simulink library "Vessel"  (R2023a)
settings: Solver=VariableStepAuto  StartTime=0.0  StopTime=10.0  RelTol=1e-3
undefined symbols (not defined in the file): A_ann_aor, alpha1, alpha2, atrium_ventricle, BSA, control, conversion_factor, DAP, DLVP, DP_close_aor, DP_open_aor, DPP, DRVP, E0, E_max, E_min, E_sa_0, E_sv_0, eta, g, K_vc_aor, K_vo_aor, l, L0, lambda, m1, m2, M_rg_aor, M_st_aor, MAP, MPP, n, P0, p_septum_on_off, p_th_on_off, phi, PVR, Q_max, rho, SAP, SI, sigma, SLVP, SPP, SRVP, SVR, t_delay, Ts, UVV_0, V0, V_0, V_max, V_tot, Y_aorta, Y_control
libraries: $bdroot x100, simulink x39, dspsigops x20, slpidlib x11, eeGeneralControl x2, dspstat3 x1
(part 3 of 4)

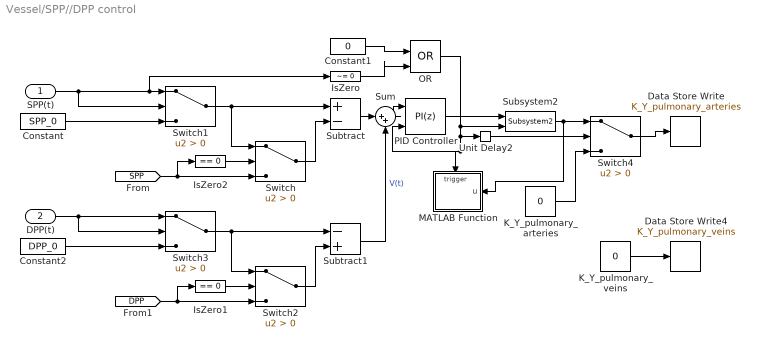
== system Vessel/SPP//DPP control ==
  SPP(t) : Inport
  DPP(t) : Inport  Port=2
  Constant : Constant  Value=SPP_0
  Constant1 : Constant  Value=0
  Constant2 : Constant  Value=DPP_0
  Data Store Write : DataStoreWrite  DataStoreName=K_Y_pulmonary_arteries  IndexOptions=Index vector (dialog)  Indices=1  OutputSizes=1
  Data Store Write4 : DataStoreWrite  DataStoreName=K_Y_pulmonary_veins  IndexOptions=Index vector (dialog)  Indices=1  OutputSizes=1
  IsZero : simulink/Logic and Bit Operations/Compare To Zero  relop=~=  OutDataTypeStr=boolean
      settings: LibrarySourceBlock=|
      | simulink/Quick Insert/Logic and Bit
      | Operations/IsZero
  IsZero1 : simulink/Logic and Bit Operations/Compare To Zero  relop===  OutDataTypeStr=boolean
      settings: LibrarySourceBlock=|
      | simulink/Quick Insert/Logic and Bit
      | Operations/IsZero
  IsZero2 : simulink/Logic and Bit Operations/Compare To Zero  relop===  OutDataTypeStr=boolean
      settings: LibrarySourceBlock=|
      | simulink/Quick Insert/Logic and Bit
      | Operations/IsZero
  K_Y_pulmonary_arteries : Constant  Value=0
  K_Y_pulmonary_veins : Constant  Value=0
  MATLAB Function : MATLAB Function  TreatAsAtomicUnit=on
  OR : Logic  Operator=OR  IconShape=distinctive  AllPortsSameDT=off  OutDataTypeStr=boolean
  PID Controller : slpidlib/PID Controller  Controller=PI  Form=Parallel  TimeDomain=Discrete-time  UseExternalTs=off  SampleTime=dt  IntegratorMethod=Forward Euler  FilterMethod=Forward Euler  ControllerParametersSource=internal  P=0.005  I=0.005  UseKiTs=off  D=0.01  N=100  UseFilter=on  TunerSelectOption=Transfer Function Based (PID Tuner App)  InitialConditionSource=internal  InitialConditionForIntegrator=0  InitialConditionForFilter=0  DifferentiatorICPrevScaledInput=0  ExternalReset=either  TrackingMode=off  Kt=1  LimitOutput=on  SatLimitsSource=internal  UpperSaturationLimit=2  LowerSaturationLimit=-0.99  LinearizeAsGain=on  AntiWindupMode=none  Kb=1  LimitIntegrator=off  UpperIntegratorSaturationLimit=inf  LowerIntegratorSaturationLimit=-inf  POutMin=[]  POutMax=[]  IOutMin=[]  IOutMax=[]  DOutMin=[]  DOutMax=[]  NOutMin=[]  NOutMax=[]  SumOutMin=[]  SumOutMax=[]  SaturationOutMin=[]  SaturationOutMax=[]  PParamMin=[]  PParamMax=[]  IParamMin=[]  IParamMax=[]  DParamMin=[]  DParamMax=[]  NParamMin=[]  NParamMax=[]  KbParamMin=[]  KbParamMax=[]  KtParamMin=[]  KtParamMax=[]  KbOutMin=[]  KbOutMax=[]  KtOutMin=[]  KtOutMax=[]  IntegratorOutMin=[]  IntegratorOutMax=[]  FilterOutMin=[]  FilterOutMax=[]  SumI1OutMin=[]  SumI1OutMax=[]  SumI2OutMin=[]  SumI2OutMax=[]  SumI3OutMin=[]  SumI3OutMax=[]  SumI4OutMin=[]  SumI4OutMax=[]  SumDOutMin=[]  SumDOutMax=[]  DifferentiatorOutMin=[]  DifferentiatorOutMax=[]  FilterDiffOutCoefMin=[]  FilterDiffOutCoefMax=[]  ReciprocalOutMin=[]  ReciprocalOutMax=[]  SumDenOutMin=[]  SumDenOutMax=[]  SumNumOutMin=[]  SumNumOutMax=[]  DivideOutMin=[]  DivideOutMax=[]  UdiffTsProdOutMin=[]  UdiffTsProdOutMax=[]  NTsProdOutMin=[]  NTsProdOutMax=[]  UintegralTsProdOutMin=[]  UintegralTsProdOutMax=[]  UngainTsProdOutMin=[]  UngainTsProdOutMax=[]  ClampingZeroOutDataTypeStr=Inherit: Inherit via back propagation  ClampingZeroOutMin=[]  ClampingZeroOutMax=[]  FilterDenConstantOutDataTypeStr=Inherit: Inherit via back propagation  FilterDenConstantOutMin=[]  FilterDenConstantOutMax=[]  PCopyOutDataTypeStr=Inherit: Inherit via back propagation  PCopyOutMin=[]  PCopyOutMax=[]  NCopyOutDataTypeStr=Inherit: Inherit via back propagation  NCopyOutMin=[]  NCopyOutMax=[]  IntegratorContinuousStateAttributes=''  IntegratorStateMustResolveToSignalObject=off  IntegratorRTWStateStorageClass=Auto  FilterContinuousStateAttributes=''  FilterStateMustResolveToSignalObject=off  FilterRTWStateStorageClass=Auto  ParallelPVariant=InternalParameters  IdealPVariant=Disabled  IVariant=InternalParameters  DVariant=Disabled  IntegratorVariant=Discrete  SatVariant=Enabled  AWVariant=Passthrough  PCopyVariant=Disabled  TRVariant=Disabled  FdbkBlocksVariant=Forward  IdealPFdbkVariant=Disabled  SatFdbkVariant=Disabled  DerivativeFilterVariant=Disabled  NVariant=Disabled  NCopyVariant=Disabled_SignalSpec  FilterICVariant=Disabled  IntegratorICVariant=InternalICs  ExternalResetVariant=ExternalReset  TRSumVariant=Passthrough  SumFdbkVariant=Disabled  SumVariant=Sum_PI  TsampFilterVariant=InternalTs  TsampNgainVariant=Passthrough  TsampIntegralVariant=Disabled_SignalSpec  ExternalSaturationOutDataTypeStr=Inherit: Same as second input
  Subsystem2 : $bdroot/SVR Control/Subsystem2  SystemSampleTime=-1  VariantActivationTime=update diagram  Latency=0  AutoFrameSizeCalculation=off
  Subtract : Sum  Inputs=+-
  Subtract1 : Sum  Inputs=-+
  Sum : Sum  Inputs=|++
  Switch{,1..4} (5 alike) : Switch  Criteria=u2 > Threshold  SaturateOnIntegerOverflow=off  InputSameDT=off
  Unit Delay2 : UnitDelay  SampleTime=-1  HasFrameUpgradeWarning=on
  wires:
  Sum/1 -> PID Controller/1
  Subtract/1 -> Sum/1
  Switch3/1 -> Subtract1/1, Switch2/1
  Constant2/1 -> Switch3/3
  Subtract1/1 -> Sum/2  "V(t)"
  IsZero1/1 -> Switch2/2
  Switch2/1 -> Subtract1/2
  DPP(t)/1 -> Switch3/2, Switch3/1
  [DPP] -> IsZero1/1, Switch2/3
  PID Controller/1 -> Subsystem2/1
  Constant1/1 -> OR/1
  IsZero/1 -> OR/2
  Switch1/1 -> Switch/1, Subtract/1
  SPP(t)/1 -> Switch1/1, IsZero/1, Switch1/2
  IsZero2/1 -> Switch/2
  Switch/1 -> Subtract/2
  [SPP] -> IsZero2/1, Switch/3
  Constant/1 -> Switch1/3
  Switch4/1 -> Data Store Write/1
  K_Y_pulmonary_veins/1 -> Data Store Write4/1
  K_Y_pulmonary_arteries/1 -> Switch4/3
  OR/1 -> Unit Delay2/1, PID Controller/2, MATLAB Function/Trigger, Subsystem2/2
  Subsystem2/1 -> Switch4/1, MATLAB Function/1(u)
  Unit Delay2/1 -> Switch4/2

== system Vessel/SRVP control ==
  SRVP(t) : Inport
  Constant : Constant  Value=SRVP_0
  Constant1 : Constant  Value=0
  Data Store Write : DataStoreWrite  DataStoreName=K_RV_Emax  IndexOptions=Index vector (dialog)  Indices=1  OutputSizes=1
  Data Store Write10 : DataStoreWrite  DataStoreName=K_RA_Emin  IndexOptions=Index vector (dialog)  Indices=1  OutputSizes=1
  Data Store Write11 : DataStoreWrite  DataStoreName=K_RV_Emin  IndexOptions=Index vector (dialog)  Indices=1  OutputSizes=1
  Data Store Write9 : DataStoreWrite  DataStoreName=K_RA_Emax  IndexOptions=Index vector (dialog)  Indices=1  OutputSizes=1
  IsZero : simulink/Logic and Bit Operations/Compare To Zero  relop=~=  OutDataTypeStr=boolean
      settings: LibrarySourceBlock=|
      | simulink/Quick Insert/Logic and Bit
      | Operations/IsZero
  IsZero2 : simulink/Logic and Bit Operations/Compare To Zero  relop===  OutDataTypeStr=boolean
      settings: LibrarySourceBlock=|
      | simulink/Quick Insert/Logic and Bit
      | Operations/IsZero
  K_RA_Emax : Constant  Value=0
  K_RA_Emin : Constant  Value=0
  K_RV_Emax : Constant  Value=0
  K_RV_Emin : Constant  Value=0
  MATLAB Function : MATLAB Function  TreatAsAtomicUnit=on
  OR : Logic  Operator=OR  IconShape=distinctive  AllPortsSameDT=off  OutDataTypeStr=boolean
  PID Controller : slpidlib/PID Controller  Controller=PI  Form=Parallel  TimeDomain=Discrete-time  UseExternalTs=off  SampleTime=dt  IntegratorMethod=Forward Euler  FilterMethod=Forward Euler  ControllerParametersSource=internal  P=0.005  I=0.005  UseKiTs=off  D=0.01  N=100  UseFilter=on  TunerSelectOption=Transfer Function Based (PID Tuner App)  InitialConditionSource=internal  InitialConditionForIntegrator=0  InitialConditionForFilter=0  DifferentiatorICPrevScaledInput=0  ExternalReset=either  TrackingMode=off  Kt=1  LimitOutput=on  SatLimitsSource=internal  UpperSaturationLimit=2  LowerSaturationLimit=-0.99  LinearizeAsGain=on  AntiWindupMode=none  Kb=1  LimitIntegrator=off  UpperIntegratorSaturationLimit=inf  LowerIntegratorSaturationLimit=-inf  POutMin=[]  POutMax=[]  IOutMin=[]  IOutMax=[]  DOutMin=[]  DOutMax=[]  NOutMin=[]  NOutMax=[]  SumOutMin=[]  SumOutMax=[]  SaturationOutMin=[]  SaturationOutMax=[]  PParamMin=[]  PParamMax=[]  IParamMin=[]  IParamMax=[]  DParamMin=[]  DParamMax=[]  NParamMin=[]  NParamMax=[]  KbParamMin=[]  KbParamMax=[]  KtParamMin=[]  KtParamMax=[]  KbOutMin=[]  KbOutMax=[]  KtOutMin=[]  KtOutMax=[]  IntegratorOutMin=[]  IntegratorOutMax=[]  FilterOutMin=[]  FilterOutMax=[]  SumI1OutMin=[]  SumI1OutMax=[]  SumI2OutMin=[]  SumI2OutMax=[]  SumI3OutMin=[]  SumI3OutMax=[]  SumI4OutMin=[]  SumI4OutMax=[]  SumDOutMin=[]  SumDOutMax=[]  DifferentiatorOutMin=[]  DifferentiatorOutMax=[]  FilterDiffOutCoefMin=[]  FilterDiffOutCoefMax=[]  ReciprocalOutMin=[]  ReciprocalOutMax=[]  SumDenOutMin=[]  SumDenOutMax=[]  SumNumOutMin=[]  SumNumOutMax=[]  DivideOutMin=[]  DivideOutMax=[]  UdiffTsProdOutMin=[]  UdiffTsProdOutMax=[]  NTsProdOutMin=[]  NTsProdOutMax=[]  UintegralTsProdOutMin=[]  UintegralTsProdOutMax=[]  UngainTsProdOutMin=[]  UngainTsProdOutMax=[]  ClampingZeroOutDataTypeStr=Inherit: Inherit via back propagation  ClampingZeroOutMin=[]  ClampingZeroOutMax=[]  FilterDenConstantOutDataTypeStr=Inherit: Inherit via back propagation  FilterDenConstantOutMin=[]  FilterDenConstantOutMax=[]  PCopyOutDataTypeStr=Inherit: Inherit via back propagation  PCopyOutMin=[]  PCopyOutMax=[]  NCopyOutDataTypeStr=Inherit: Inherit via back propagation  NCopyOutMin=[]  NCopyOutMax=[]  IntegratorContinuousStateAttributes=''  IntegratorStateMustResolveToSignalObject=off  IntegratorRTWStateStorageClass=Auto  FilterContinuousStateAttributes=''  FilterStateMustResolveToSignalObject=off  FilterRTWStateStorageClass=Auto  ParallelPVariant=InternalParameters  IdealPVariant=Disabled  IVariant=InternalParameters  DVariant=Disabled  IntegratorVariant=Discrete  SatVariant=Enabled  AWVariant=Passthrough  PCopyVariant=Disabled  TRVariant=Disabled  FdbkBlocksVariant=Forward  IdealPFdbkVariant=Disabled  SatFdbkVariant=Disabled  DerivativeFilterVariant=Disabled  NVariant=Disabled  NCopyVariant=Disabled_SignalSpec  FilterICVariant=Disabled  IntegratorICVariant=InternalICs  ExternalResetVariant=ExternalReset  TRSumVariant=Passthrough  SumFdbkVariant=Disabled  SumVariant=Sum_PI  TsampFilterVariant=InternalTs  TsampNgainVariant=Passthrough  TsampIntegralVariant=Disabled_SignalSpec  ExternalSaturationOutDataTypeStr=Inherit: Same as second input
  Subsystem2 : $bdroot/SVR Control/Subsystem2  SystemSampleTime=-1  VariantActivationTime=update diagram  Latency=0  AutoFrameSizeCalculation=off
  Subtract : Sum  Inputs=+-
  Switch : Switch  Criteria=u2 > Threshold  SaturateOnIntegerOverflow=off  InputSameDT=off
  Switch1 : Switch  Criteria=u2 > Threshold  SaturateOnIntegerOverflow=off  InputSameDT=off
  Switch2 : Switch  Criteria=u2 > Threshold  SaturateOnIntegerOverflow=off  InputSameDT=off
  Unit Delay2 : UnitDelay  SampleTime=-1  HasFrameUpgradeWarning=on
  wires:
  Subtract/1 -> PID Controller/1  "V(t)"
  Constant/1 -> Switch1/3
  [MPP] -> IsZero2/1, Switch/3
  Switch/1 -> Subtract/2
  IsZero2/1 -> Switch/2
  SRVP(t)/1 -> Switch1/2, IsZero/1, Switch1/1
  Switch1/1 -> Subtract/1, Switch/1
  IsZero/1 -> OR/2
  Constant1/1 -> OR/1
  PID Controller/1 -> Subsystem2/1
  K_RA_Emin/1 -> Data Store Write10/1
  K_RV_Emax/1 -> Switch2/3
  K_RV_Emin/1 -> Data Store Write11/1
  K_RA_Emax/1 -> Data Store Write9/1
  Switch2/1 -> Data Store Write/1
  OR/1 -> PID Controller/2, MATLAB Function/Trigger, Unit Delay2/1, Subsystem2/2
  Subsystem2/1 -> MATLAB Function/1(u), Switch2/1
  Unit Delay2/1 -> Switch2/2

== system Vessel/SVR Control ==
  SVR(t) : Inport
  Constant : Constant  Value=SVR_0
  Constant1 : Constant  Value=0
  Data Store Write : DataStoreWrite  DataStoreName=K_svr  IndexOptions=Index vector (dialog)  Indices=1  OutputSizes=1
  IsZero : simulink/Logic and Bit Operations/Compare To Zero  relop=~=  OutDataTypeStr=boolean
      settings: LibrarySourceBlock=|
      | simulink/Quick Insert/Logic and Bit
      | Operations/IsZero
  K_svr : Constant  Value=0
  MATLAB Function : MATLAB Function  TreatAsAtomicUnit=on
  OR : Logic  Operator=OR  IconShape=distinctive  AllPortsSameDT=off  OutDataTypeStr=boolean
  PID Controller : slpidlib/PID Controller  Controller=PI  Form=Parallel  TimeDomain=Continuous-time  UseExternalTs=off  SampleTime=-1  IntegratorMethod=Forward Euler  FilterMethod=Forward Euler  ControllerParametersSource=internal  P=0.2  I=0.2  UseKiTs=off  D=0.01  N=100  UseFilter=on  TunerSelectOption=Transfer Function Based (PID Tuner App)  InitialConditionSource=internal  InitialConditionForIntegrator=0  InitialConditionForFilter=0  DifferentiatorICPrevScaledInput=0  ExternalReset=either  TrackingMode=off  Kt=1  LimitOutput=off  SatLimitsSource=internal  UpperSaturationLimit=inf  LowerSaturationLimit=-inf  LinearizeAsGain=on  AntiWindupMode=none  Kb=1  LimitIntegrator=off  UpperIntegratorSaturationLimit=inf  LowerIntegratorSaturationLimit=-inf  POutMin=[]  POutMax=[]  IOutMin=[]  IOutMax=[]  DOutMin=[]  DOutMax=[]  NOutMin=[]  NOutMax=[]  SumOutMin=[]  SumOutMax=[]  SaturationOutMin=[]  SaturationOutMax=[]  PParamMin=[]  PParamMax=[]  IParamMin=[]  IParamMax=[]  DParamMin=[]  DParamMax=[]  NParamMin=[]  NParamMax=[]  KbParamMin=[]  KbParamMax=[]  KtParamMin=[]  KtParamMax=[]  KbOutMin=[]  KbOutMax=[]  KtOutMin=[]  KtOutMax=[]  IntegratorOutMin=[]  IntegratorOutMax=[]  FilterOutMin=[]  FilterOutMax=[]  SumI1OutMin=[]  SumI1OutMax=[]  SumI2OutMin=[]  SumI2OutMax=[]  SumI3OutMin=[]  SumI3OutMax=[]  SumI4OutMin=[]  SumI4OutMax=[]  SumDOutMin=[]  SumDOutMax=[]  DifferentiatorOutMin=[]  DifferentiatorOutMax=[]  FilterDiffOutCoefMin=[]  FilterDiffOutCoefMax=[]  ReciprocalOutMin=[]  ReciprocalOutMax=[]  SumDenOutMin=[]  SumDenOutMax=[]  SumNumOutMin=[]  SumNumOutMax=[]  DivideOutMin=[]  DivideOutMax=[]  UdiffTsProdOutMin=[]  UdiffTsProdOutMax=[]  NTsProdOutMin=[]  NTsProdOutMax=[]  UintegralTsProdOutMin=[]  UintegralTsProdOutMax=[]  UngainTsProdOutMin=[]  UngainTsProdOutMax=[]  ClampingZeroOutDataTypeStr=Inherit: Inherit via back propagation  ClampingZeroOutMin=[]  ClampingZeroOutMax=[]  FilterDenConstantOutDataTypeStr=Inherit: Inherit via back propagation  FilterDenConstantOutMin=[]  FilterDenConstantOutMax=[]  PCopyOutDataTypeStr=Inherit: Inherit via back propagation  PCopyOutMin=[]  PCopyOutMax=[]  NCopyOutDataTypeStr=Inherit: Inherit via back propagation  NCopyOutMin=[]  NCopyOutMax=[]  IntegratorContinuousStateAttributes=''  IntegratorStateMustResolveToSignalObject=off  IntegratorRTWStateStorageClass=Auto  FilterContinuousStateAttributes=''  FilterStateMustResolveToSignalObject=off  FilterRTWStateStorageClass=Auto  ParallelPVariant=InternalParameters  IdealPVariant=Disabled  IVariant=InternalParameters  DVariant=Disabled  IntegratorVariant=Continuous  SatVariant=Disabled  AWVariant=Passthrough  PCopyVariant=Disabled  TRVariant=Disabled  FdbkBlocksVariant=Forward  IdealPFdbkVariant=Disabled  SatFdbkVariant=Disabled  DerivativeFilterVariant=Disabled  NVariant=Disabled  NCopyVariant=Disabled_SignalSpec  FilterICVariant=Disabled  IntegratorICVariant=InternalICs  ExternalResetVariant=ExternalReset  TRSumVariant=Passthrough  SumFdbkVariant=Disabled  SumVariant=Sum_PI  TsampFilterVariant=InternalTs  TsampNgainVariant=Passthrough  TsampIntegralVariant=Disabled_SignalSpec  ExternalSaturationOutDataTypeStr=Inherit: Same as second input
  Subsystem1 : Subsystem
  Subsystem2 : Subsystem
  Subtract : Sum  Inputs=-+
  Switch : Switch  Criteria=u2 > Threshold  SaturateOnIntegerOverflow=off  InputSameDT=off
  Switch1 : Switch  Criteria=u2 > Threshold  SaturateOnIntegerOverflow=off  InputSameDT=off
  Switch2 : Switch  Criteria=u2 > Threshold  SaturateOnIntegerOverflow=off  InputSameDT=off
  Unit Delay : UnitDelay  SampleTime=-1  HasFrameUpgradeWarning=on
  wires:
  Subtract/1 -> PID Controller/1  "V(t)"
  Constant/1 -> Switch1/3
  [SVR] -> Subsystem1/1(In1), Switch/3
  Switch/1 -> Subtract/2
  Subsystem1/1(Out1) -> Switch/2
  SVR(t)/1 -> Switch1/2, IsZero/1, Switch1/1
  Switch1/1 -> Subtract/1, Switch/1
  IsZero/1 -> OR/2
  Constant1/1 -> OR/1
  Switch2/1 -> Data Store Write/1
  K_svr/1 -> Switch2/3
  OR/1 -> Subsystem2/2(Trigger), Unit Delay/1, PID Controller/2, MATLAB Function/Trigger
  PID Controller/1 -> Subsystem2/1(Signal)
  Subsystem2/1(Out) -> MATLAB Function/1(u), Switch2/1
  Unit Delay/1 -> Switch2/2

== system Vessel/Systolic Pressure ==
  P_in : Inport
  MinMax Running Resettable1 : simulink/Math Operations/MinMax Running Resettable  Function=max  vinit=0
      settings: AttributesFormatString=%<vinit>
  Pulse Generator1 : DiscretePulseGenerator  PulseType=Time based  TimeSource=Use external signal  Period=100  PulseWidth=1e-3
  Sample and Hold1 : dspsigops/Sample and Hold  trig=Rising edge  initCond=0  latchinput=on
  P_sys : Outport
  wires:
  MinMax Running Resettable1/1 -> Sample and Hold1/1
  Pulse Generator1/1 -> MinMax Running Resettable1/2, Sample and Hold1/Trigger
  Sample and Hold1/1 -> P_sys/1
  P_in/1 -> MinMax Running Resettable1/1
  [t_b] -> Pulse Generator1/1

== system Vessel/Time varying elastance (old) ==
  v_ed : Inport
  V : Inport  Port=2
  V' : Inport  Port=3
  Constant : Constant  Value=m1
  Constant1 : Constant  Value=m2
  Constant10 : Constant  Value=alpha2
  Constant12 : Constant  Value=Q_max
  Constant2 : Constant  Value=t_delay
  Constant4 : Constant  Value=E_max
  Constant5 : Constant  Value=E_min
  Constant6 : Constant  Value=sigma
  Constant7 : Constant  Value=alpha1
  Constant8 : Constant  Value=V_0
  Constant9 : Constant  Value=V_max
  Data Store Read : DataStoreRead  DataStoreName=T  IndexOptions=Index vector (dialog)  Indices=1  OutputSizes=1
  Data Store Read1 : DataStoreRead  DataStoreName=T  IndexOptions=Index vector (dialog)  Indices=1  OutputSizes=1
  Display : Display
  Display1 : Display
  MATLAB Function : MATLAB Function  TreatAsAtomicUnit=on
  Product : Product
  Sqrt : Sqrt
  E(t) : Outport
  wires:
  MATLAB Function/1(E) -> E(t)/1  "E(t)"
  Constant12/1 -> MATLAB Function/14(Q_max)
  v_ed/1 -> MATLAB Function/15(v_ed)
  V'/1 -> MATLAB Function/13(q)
  Constant9/1 -> MATLAB Function/12(V_max)
  Constant5/1 -> MATLAB Function/6(E_min)
  V/1 -> MATLAB Function/11(V)
  Constant8/1 -> MATLAB Function/10(V_0)
  Constant6/1 -> MATLAB Function/9(sigma)
  Data Store Read/1 -> MATLAB Function/8(T)
  Constant7/1 -> MATLAB Function/3(alpha1_ref)
  Constant/1 -> MATLAB Function/1(m1_ref)
  Constant4/1 -> MATLAB Function/5(E_max)
  [t_b] -> MATLAB Function/7(t)
  Constant1/1 -> MATLAB Function/2(m2_ref)
  Constant10/1 -> MATLAB Function/4(alpha2_ref)
  MATLAB Function/2(e_min) -> Display/1
  MATLAB Function/3(e_max) -> Display1/1
  Sqrt/1 -> Product/2
  Product/1 -> MATLAB Function/16(t_delay)
  Constant2/1 -> Product/1
  Data Store Read1/1 -> Sqrt/1

== system Vessel/Time varying elastance1 ==
  v_ed : Inport
  V : Inport  Port=2
  V' : Inport  Port=3
  Add : Sum
  Product : Product
  Subsystem : Subsystem
  e_max : Subsystem
  e_min : Subsystem
  k : Subsystem
  E(t) : Outport
  wires:
  Add/1 -> E(t)/1  "E(t)"
  e_max/1(e_max) -> k/3(e_max)
  Subsystem/2("f(g1, g2, t-t_delay)") -> Product/2
  k/1(k) -> Product/1
  Product/1 -> Add/1
  [t_b] -> Subsystem/1(t), k/1(t)
  V/1 -> e_min/1(V)
  e_min/1(e_min) -> Add/2, k/4(e_min)
  V'/1 -> e_max/2(V')
  v_ed/1 -> e_max/1(v_ed)
  Subsystem/1("f(g1, g2)") -> k/2("f(g1, g2)")

== system Vessel/Total Pulmonary resistance ==
  P_pu : Inport
  P_LA : Inport  Port=2
  Abs : Abs  SaturateOnIntegerOverflow=off
  Divide : Product  Inputs=*/
  Gain : Gain  Gain=60
  MAP1 : $bdroot/MAP  SystemSampleTime=-1  VariantActivationTime=update diagram  Latency=0  AutoFrameSizeCalculation=off
  Subtract1 : Sum  Inputs=-+
  tag scope: PVR=global
  wires:
  Abs/1 -> Gain/1
  Divide/1 -> Abs/1
  Subtract1/1 -> MAP1/1
  [CO] -> Divide/2
  P_LA/1 -> Subtract1/2
  Gain/1 -> [PVR]
  P_pu/1 -> Subtract1/1
  MAP1/1 -> Divide/1

== system Vessel/Total Systemic Resistance ==
  P_ao : Inport
  P_RA : Inport  Port=2
  Abs1 : Abs  SaturateOnIntegerOverflow=off
  Divide1 : Product  Inputs=*/
  Gain : Gain  Gain=60
  MAP1 : $bdroot/MAP  SystemSampleTime=-1  VariantActivationTime=update diagram  Latency=0  AutoFrameSizeCalculation=off
  Subtract1 : Sum  Inputs=+-
  tag scope: SVR=global
  wires:
  Abs1/1 -> Gain/1
  P_ao/1 -> Subtract1/1
  Divide1/1 -> Abs1/1
  Subtract1/1 -> MAP1/1
  P_RA/1 -> Subtract1/2
  [CO] -> Divide1/2
  Gain/1 -> [SVR]
  MAP1/1 -> Divide1/1

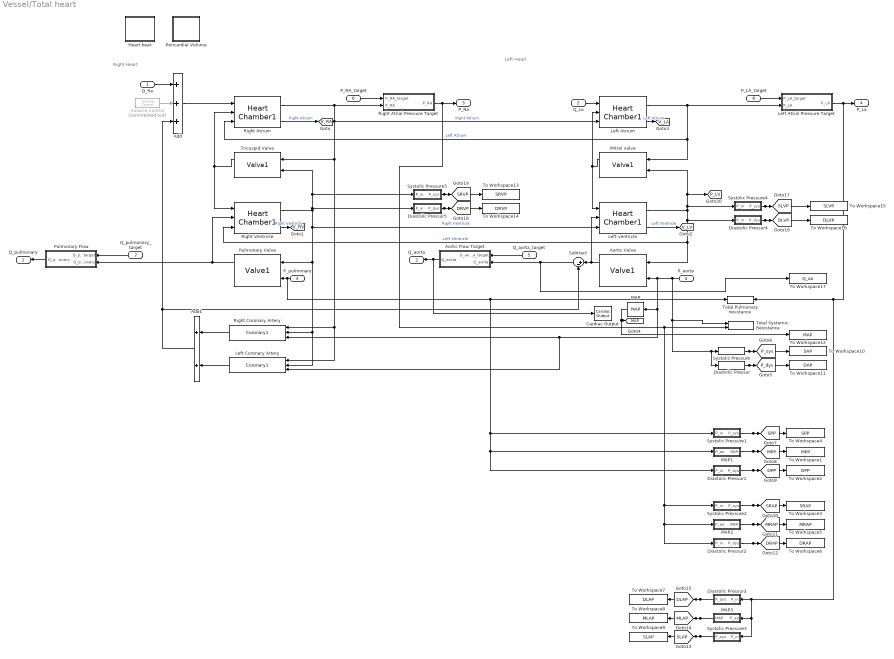
== system Vessel/Total heart ==
  note: Left Heart
  note: Right Heart
  Q_Ra : Inport
  Q_La : Inport  Port=2
  P_pulmonary : Inport  Port=3
  P_aorta : Inport  Port=4
  Q_aorta_target : Inport  Port=5
  P_RA_target : Inport  Port=6
  Q_pulmonary_target : Inport  Port=7
  P_LA_target : Inport  Port=8
  Add : Sum  Inputs=+++
  Add1 : Sum
  Aortic Flow Target : Subsystem
  Aortic Valve : $bdroot/Valve1  A_ann=A_ann_aor  K_vo=K_vo_aor  K_vc=K_vc_aor  M_st=M_st_aor  M_rg=M_rg_aor  DP_open=DP_open_aor  DP_close=DP_close_aor  Q_max=Q_max_lv  Q_min=-1000
  Cardiac Output : $bdroot/Cardiac Output  SystemSampleTime=-1  VariantActivationTime=update diagram  Latency=0  AutoFrameSizeCalculation=off
  Diastolic Pressur : $bdroot/Diastolic Pressur  SystemSampleTime=-1  VariantActivationTime=update diagram  Latency=0  AutoFrameSizeCalculation=off
  Diastolic Pressur1 : Subsystem
  Diastolic Pressur2 : Subsystem
  Diastolic Pressur3 : Subsystem
  Diastolic Pressur4 : Subsystem
  Diastolic Pressur5 : Subsystem
  Heart beat : Subsystem
  Left Atrial Pressure Target : Subsystem
  Left Atrium : $bdroot/Heart Chamber1  control=Left Atrium  E_max=E_max_la  E_min=E_min_la  alpha1=alpha1_la  alpha2=alpha2_la  m1=m1_la  m2=m2_la  R_wall=R_wall_la  t_delay=t_delay_la  V_0=V_0_la  v_o=v_o_la  sigma=sigma_la  V_max=V_max_la  Q_max=Q_max_la  T0=T0  P_pc_0=P_pc_0  K_pc=K_pc  V_pc_0=V_pc_0  V_pe=V_pe  phi_pc=phi_pc  E_sa_0=E_sa_0  E_sv_0=E_sv_0  atrium_ventricle=Atrium
  Left Coronary Artery : $bdroot/Coronary1  R_ca=R_lca
  Left ventricle : $bdroot/Heart Chamber1  control=Left Ventricle  E_max=E_max_lv  E_min=E_min_lv  alpha1=alpha1_lv  alpha2=alpha2_lv  m1=m1_lv  m2=m2_lv  R_wall=R_wall_lv  t_delay=t_delay_lv  V_0=V_0_lv  v_o=v_o_lv  sigma=sigma_lv  V_max=V_max_lv  Q_max=Q_max_lv  T0=T0  P_pc_0=P_pc_0  K_pc=K_pc  V_pc_0=V_pc_0  V_pe=V_pe  phi_pc=phi_pc  E_sa_0=E_sa_0  E_sv_0=E_sv_0  atrium_ventricle=Ventricle
  MAP : $bdroot/MAP  SystemSampleTime=-1  VariantActivationTime=update diagram  Latency=0  AutoFrameSizeCalculation=off
  MAP1 : Subsystem
  MAP2 : Subsystem
  MAP3 : Subsystem
  Mitral valve : $bdroot/Valve1  A_ann=A_ann_mit  K_vo=K_vo_mit  K_vc=K_vc_mit  M_st=M_st_mit  M_rg=M_rg_mit  DP_open=DP_open_mit  DP_close=DP_close_mit  Q_max=Q_max_la  Q_min=-1000
  Pericardial Volume : Subsystem
  Pulmonary Flow : Subsystem
  Pulmonary Valve : $bdroot/Valve1  A_ann=A_ann_pul  K_vo=K_vo_pul  K_vc=K_vc_pul  M_st=M_st_pul  M_rg=M_rg_pul  DP_open=DP_open_pul  DP_close=DP_close_pul  Q_max=Q_max_rv  Q_min=-1000
  Right Atrial Pressure Target : Subsystem
  Right Atrium : $bdroot/Heart Chamber1  control=Right Atrium  E_max=E_max_ra  E_min=E_min_ra  alpha1=alpha1_ra  alpha2=alpha2_ra  m1=m1_ra  m2=m2_ra  R_wall=R_wall_ra  t_delay=t_delay_ra  V_0=V_0_ra  v_o=v_o_ra  sigma=sigma_ra  V_max=V_max_ra  Q_max=Q_max_ra  T0=T0  P_pc_0=P_pc_0  K_pc=K_pc  V_pc_0=V_pc_0  V_pe=V_pe  phi_pc=phi_pc  E_sa_0=E_sa_0  E_sv_0=E_sv_0  atrium_ventricle=Atrium
  Right Coronary Artery : $bdroot/Coronary1  R_ca=R_rca
  Right Ventricle : $bdroot/Heart Chamber1  control=Right Ventricle  E_max=E_max_rv  E_min=E_min_rv  alpha1=alpha1_rv  alpha2=alpha2_rv  m1=m1_rv  m2=m2_rv  R_wall=R_wall_rv  t_delay=t_delay_rv  V_0=V_0_rv  v_o=v_o_rv  sigma=sigma_rv  V_max=V_max_rv  Q_max=Q_max_rv  T0=T0  P_pc_0=P_pc_0  K_pc=K_pc  V_pc_0=V_pc_0  V_pe=V_pe  phi_pc=phi_pc  E_sa_0=E_sa_0  E_sv_0=E_sv_0  atrium_ventricle=Ventricle
  Subtract : Sum  Inputs=|+-
  Systolic Pressure : $bdroot/Systolic Pressure  SystemSampleTime=-1  VariantActivationTime=update diagram  Latency=0  AutoFrameSizeCalculation=off
  Systolic Pressure1 : Subsystem
  Systolic Pressure2 : Subsystem
  Systolic Pressure3 : Subsystem
  Systolic Pressure4 : Subsystem
  Systolic Pressure5 : Subsystem
  To Workspace1 : ToWorkspace  VariableName=MPP  SampleTime=-1
  To Workspace10 : ToWorkspace  VariableName=SAP  SampleTime=-1
  To Workspace11 : ToWorkspace  VariableName=DAP  SampleTime=-1
  To Workspace12 : ToWorkspace  VariableName=MAP  SampleTime=-1
  To Workspace13 : ToWorkspace  VariableName=SRVP  SampleTime=-1
  To Workspace14 : ToWorkspace  VariableName=DRVP  SampleTime=-1
  To Workspace15 : ToWorkspace  VariableName=SLVP  SampleTime=-1
  To Workspace16 : ToWorkspace  VariableName=DLVP  SampleTime=-1
  To Workspace17 : ToWorkspace  VariableName=Q_ao  SampleTime=-1
  To Workspace2 : ToWorkspace  VariableName=DPP  SampleTime=-1
  To Workspace3 : ToWorkspace  VariableName=SRAP  SampleTime=-1
  To Workspace4 : ToWorkspace  VariableName=SPP  SampleTime=-1
  To Workspace5 : ToWorkspace  VariableName=MRAP  SampleTime=-1
  To Workspace6 : ToWorkspace  VariableName=DRAP  SampleTime=-1
  To Workspace7 : ToWorkspace  VariableName=DLAP  SampleTime=-1
  To Workspace8 : ToWorkspace  VariableName=MLAP  SampleTime=-1
  To Workspace9 : ToWorkspace  VariableName=SLAP  SampleTime=-1
  Total Pulmonary resistance : $bdroot/Total Pulmonary resistance  SystemSampleTime=-1  VariantActivationTime=update diagram  Latency=0  AutoFrameSizeCalculation=off
      settings: PortSchema="{\"entries\":[{\"content\":{\"sides\":[{\"content\":{\"connectorIds\":[\"In1\"]},\"type\":\"ConnectorPlacement.EquallySpacedRectSide\",\"uuid\":\"c9341461-c171-4eac-a287-36e7cd79ba9c\"},{\"content\":{\"connectorIds\":[\"In2\"],\"side\":\"RIGHT\"},\"type\":\"ConnectorPlacement.EquallySpacedRectSide\",\"uuid\":\"dd479575-dfa7-40be-8840-552306c7a812\"},{\"content\":{\"connectorIds\":[],\"side\":\"TOP\"},\"type\":\"ConnectorPlacement.EquallySpacedRectSide\",\"uuid\":\"55fb924b-6719-416a-80e5-0f49fb901268\"}]},\"type\":\"ConnectorPlacement.EquallySpacedConnector\",\"uuid\":\"ed4dd8c3-ddc7-4a34-b37b-80f1af9032bf\"}],\"packageUris\":[\"http://schema.mathworks.com/mf0/Connector/R2020b\"],\"version\":\"1.0\"}"
  Total Systemic Resistance : $bdroot/Total Systemic Resistance  SystemSampleTime=-1  VariantActivationTime=update diagram  Latency=0  AutoFrameSizeCalculation=off
  Tricuspid Valve : $bdroot/Valve1  A_ann=A_ann_tri  K_vo=K_vo_tri  K_vc=K_vc_tri  M_st=M_st_tri  M_rg=M_rg_tri  DP_open=DP_open_tri  DP_close=DP_close_tri  Q_max=Q_max_ra  Q_min=-1000
  Volume Control : $bdroot/Volume Control  Commented=on  V_tot_0=V_tot
  Q_pulmonary : Outport
  Q_aorta : Outport  Port=2
  P_Ra : Outport  Port=3
  P_La : Outport  Port=4
  tag scope: DLAP=global, DLVP=global, DPP=global, DRAP=global, DRVP=global, MAP=global, MLAP=global, MPP=global, MRAP=global, P_LV=global, P_dys=global, P_sys=global, SLAP=global, SLVP=global, SPP=global, SRAP=global, SRVP=global, V_LA=global, V_LV=global, V_RA=global, V_RV=global
  wires:
  Q_Ra/1 -> Add/1
  Tricuspid Valve/1 -> Right Ventricle/1, Right Atrium/2
  Right Ventricle/1 -> Right Coronary Artery/2, Left Coronary Artery/2, Pulmonary Valve/1, Left ventricle/3, Systolic Pressure5/1(P_in), Tricuspid Valve/2, Diastolic Pressur5/1(P_in)  "Right Ventricle"
  Pulmonary Valve/1 -> Right Ventricle/2, Pulmonary Flow/2("Q_pulmonary ")
  Q_La/1 -> Left Atrium/1
  Mitral valve/1 -> Left ventricle/1, Left Atrium/2
  Aortic Valve/1 -> Subtract/1, Left ventricle/2
  Left Atrium/1 -> Left Atrial Pressure Target/2("P_LA "), Mitral valve/1, Right Atrium/3  "Left Atrium"
  P_aorta/1 -> Diastolic Pressur/1, Systolic Pressure/1, Total Systemic Resistance/1, Left Coronary Artery/3, Right Coronary Artery/3, MAP/1, Aortic Valve/2
  Right Atrium/2 -> [V_RA]  "Right Atrium"
  Right Ventricle/2 -> [V_RV]  "Right Ventricle"
  Left Atrium/2 -> [V_LA]  "Left Atrium"
  Left ventricle/2 -> [V_LV]  "Left Ventricle"
  Left ventricle/1 -> [P_LV], Mitral valve/2, Systolic Pressure4/1(P_in), Right Ventricle/3, Aortic Valve/1, Diastolic Pressur4/1(P_in)  "Left Ventricle"
  Right Atrium/1 -> Right Atrial Pressure Target/2("P_RA "), Tricuspid Valve/1, Left Coronary Artery/1, Right Coronary Artery/1, Left Atrium/3  "Right Atrium"
  Add/1 -> Right Atrium/1
  Right Coronary Artery/1 -> Add1/1
  Add1/1 -> Subtract/2, Add/3
  Subtract/1 -> To Workspace17/1, Aortic Flow Target/2("Q_aorta ")
  Volume Control/1 -> Add/2
  Left Coronary Artery/1 -> Add1/2
  MAP/1 -> To Workspace12/1, [MAP]
  Q_aorta_target/1 -> Aortic Flow Target/1(Q_aorta_target)
  Aortic Flow Target/1(Q_aorta) -> Cardiac Output/1, Q_aorta/1
  Right Atrial Pressure Target/1(P_RA) -> P_Ra/1, Diastolic Pressur2/1(P_in), MAP2/1(P_ao), Systolic Pressure2/1(P_in), Total Systemic Resistance/2
  P_RA_target/1 -> Right Atrial Pressure Target/1(P_RA_target)
  Pulmonary Flow/1(Q_pulmonary) -> Q_pulmonary/1
  Q_pulmonary_target/1 -> Pulmonary Flow/1(Q_pulmonary_target)
  P_LA_target/1 -> Left Atrial Pressure Target/1(P_LA_target)
  Systolic Pressure/1 -> To Workspace10/1, [P_sys]
  Systolic Pressure1/1(P_sys) -> To Workspace4/1, [SPP]
  Diastolic Pressur1/1(P_dys) -> To Workspace2/1, [DPP]
  MAP1/1(MAP) -> To Workspace1/1, [MPP]
  P_pulmonary/1 -> Diastolic Pressur1/1(P_in), MAP1/1(P_ao), Systolic Pressure1/1(P_in), Total Pulmonary resistance/1, Pulmonary Valve/2
  MAP2/1(MAP) -> To Workspace5/1, [MRAP]
  Diastolic Pressur2/1(P_dys) -> To Workspace6/1, [DRAP]
  Systolic Pressure2/1(P_sys) -> To Workspace3/1, [SRAP]
  Systolic Pressure3/1(P_sys) -> To Workspace9/1, [SLAP]
  Diastolic Pressur3/1(P_dys) -> To Workspace7/1, [DLAP]
  Left Atrial Pressure Target/1(P_LA) -> Diastolic Pressur3/1(P_in), MAP3/1(P_ao), Systolic Pressure3/1(P_in), Total Pulmonary resistance/2, P_La/1
  Systolic Pressure4/1(P_sys) -> To Workspace15/1, [SLVP]
  Diastolic Pressur4/1(P_dys) -> To Workspace16/1, [DLVP]
  Systolic Pressure5/1(P_sys) -> To Workspace13/1, [SRVP]
  Diastolic Pressur5/1(P_dys) -> To Workspace14/1, [DRVP]
  MAP3/1(MAP) -> To Workspace8/1, [MLAP]
  Diastolic Pressur/1 -> To Workspace11/1, [P_dys]

== system Vessel/Transeptal pressure ==
  V(t)-V(0) : Inport
  E(t) : Inport  Port=2
  P_chamber_other : Inport  Port=3
  Add : Sum
  Constant2 : Constant  Value=E_sv_0
  Constant3 : Constant  Value=E_sa_0
  Divide : Product  Inputs=*/
  Divide1 : Product  Inputs=***
  Divide2 : Product  Inputs=*/
  Divide3 : Product  Inputs=**
  Divide4 : Product  Inputs=**
  Subsystem : Subsystem
  Sum : Sum  Inputs=++|
  Switch : Switch  Criteria=u2 > Threshold  SaturateOnIntegerOverflow=off  InputSameDT=off
  P_chamber_this : Outport
  wires:
  Divide4/1 -> Divide/1, Sum/1  "E_sv(t)"
  Sum/1 -> Divide2/2, Divide/2
  V(t)-V(0)/1 -> Divide1/1
  Divide/1 -> Divide1/2
  E(t)/1 -> Divide4/2, Divide2/1, Divide1/3, Sum/2
  Divide2/1 -> Divide3/2
  P_chamber_other/1 -> Divide3/1
  Divide1/1 -> Add/1
  Divide3/1 -> Add/2
  Add/1 -> P_chamber_this/1
  Subsystem/1(Out1) -> Switch/2
  Constant3/1 -> Switch/1
  Constant2/1 -> Switch/3
  Switch/1 -> Divide4/1

== system Vessel/Transmural Pressure ==
  V-V0 : Inport
  Constant : Constant  Value=E0
  Constant8 : Constant  Value=P0
  Divide : Product  Inputs=*/
  Gain_Y : $bdroot/Gain_Y  SystemSampleTime=-1  VariantActivationTime=update diagram  Latency=0  AutoFrameSizeCalculation=off
  Math Function : Math
  Product6 : Product  Inputs=*/
  Product8 : Product
  P_c : Outport
  wires:
  Math Function/1 -> Product8/1
  Product6/1 -> Math Function/1
  V-V0/1 -> Product6/1
  Divide/1 -> Product6/2
  Product8/1 -> P_c/1  "P_c"
  Constant/1 -> Gain_Y/1  "E0"
  Constant8/1 -> Product8/2, Divide/1
  Gain_Y/1 -> Divide/2  "E0"

== system Vessel/Transport delay (old) ==
  In1 : Inport
  Constant1 : Constant  Value=t_delay
  Data Store Read : DataStoreRead  DataStoreName=T  IndexOptions=Index vector (dialog)  Indices=1  OutputSizes=1
  Product : Product
  Sqrt : Sqrt
  Variable Transport Delay : VariableTransportDelay  VariableDelayType=Variable transport delay  MaximumDelay=10  InitialOutput=E_min
  Out1 : Outport
  wires:
  Variable Transport Delay/1 -> Out1/1
  Product/1 -> Variable Transport Delay/2
  In1/1 -> Variable Transport Delay/1
  Constant1/1 -> Product/1
  Data Store Read/1 -> Sqrt/1
  Sqrt/1 -> Product/2

== system Vessel/UVV Control ==
  UVV(t) : Inport
  Constant : Constant  Value=UVV_0
  Constant1 : Constant  Value=0
  Data Store Write : DataStoreWrite  DataStoreName=K_uvv  IndexOptions=Index vector (dialog)  Indices=1  OutputSizes=1
  IsZero1 : simulink/Logic and Bit Operations/Compare To Zero  relop=~=  OutDataTypeStr=boolean
      settings: LibrarySourceBlock=|
      | simulink/Quick Insert/Logic and Bit
      | Operations/IsZero
  K_uvv : Constant  Value=0
  MATLAB Function : MATLAB Function  TreatAsAtomicUnit=on
  OR : Logic  Operator=OR  IconShape=distinctive  AllPortsSameDT=off  OutDataTypeStr=boolean
  PID Controller1 : slpidlib/PID Controller  Controller=PI  Form=Ideal  TimeDomain=Continuous-time  UseExternalTs=off  SampleTime=0.1  IntegratorMethod=Forward Euler  FilterMethod=Forward Euler  ControllerParametersSource=internal  P=0.2  I=0.2  UseKiTs=off  D=0.01  N=100  UseFilter=on  TunerSelectOption=Transfer Function Based (PID Tuner App)  InitialConditionSource=internal  InitialConditionForIntegrator=0  InitialConditionForFilter=0  DifferentiatorICPrevScaledInput=0  ExternalReset=either  TrackingMode=off  Kt=1  LimitOutput=on  SatLimitsSource=internal  UpperSaturationLimit=3  LowerSaturationLimit=-0.99  LinearizeAsGain=on  AntiWindupMode=none  Kb=1  LimitIntegrator=off  UpperIntegratorSaturationLimit=inf  LowerIntegratorSaturationLimit=-inf  POutMin=[]  POutMax=[]  IOutMin=[]  IOutMax=[]  DOutMin=[]  DOutMax=[]  NOutMin=[]  NOutMax=[]  SumOutMin=[]  SumOutMax=[]  SaturationOutMin=[]  SaturationOutMax=[]  PParamMin=[]  PParamMax=[]  IParamMin=[]  IParamMax=[]  DParamMin=[]  DParamMax=[]  NParamMin=[]  NParamMax=[]  KbParamMin=[]  KbParamMax=[]  KtParamMin=[]  KtParamMax=[]  KbOutMin=[]  KbOutMax=[]  KtOutMin=[]  KtOutMax=[]  IntegratorOutMin=[]  IntegratorOutMax=[]  FilterOutMin=[]  FilterOutMax=[]  SumI1OutMin=[]  SumI1OutMax=[]  SumI2OutMin=[]  SumI2OutMax=[]  SumI3OutMin=[]  SumI3OutMax=[]  SumI4OutMin=[]  SumI4OutMax=[]  SumDOutMin=[]  SumDOutMax=[]  DifferentiatorOutMin=[]  DifferentiatorOutMax=[]  FilterDiffOutCoefMin=[]  FilterDiffOutCoefMax=[]  ReciprocalOutMin=[]  ReciprocalOutMax=[]  SumDenOutMin=[]  SumDenOutMax=[]  SumNumOutMin=[]  SumNumOutMax=[]  DivideOutMin=[]  DivideOutMax=[]  UdiffTsProdOutMin=[]  UdiffTsProdOutMax=[]  NTsProdOutMin=[]  NTsProdOutMax=[]  UintegralTsProdOutMin=[]  UintegralTsProdOutMax=[]  UngainTsProdOutMin=[]  UngainTsProdOutMax=[]  ClampingZeroOutDataTypeStr=Inherit: Inherit via back propagation  ClampingZeroOutMin=[]  ClampingZeroOutMax=[]  FilterDenConstantOutDataTypeStr=Inherit: Inherit via back propagation  FilterDenConstantOutMin=[]  FilterDenConstantOutMax=[]  PCopyOutDataTypeStr=Inherit: Inherit via back propagation  PCopyOutMin=[]  PCopyOutMax=[]  NCopyOutDataTypeStr=Inherit: Inherit via back propagation  NCopyOutMin=[]  NCopyOutMax=[]  IntegratorContinuousStateAttributes=''  IntegratorStateMustResolveToSignalObject=off  IntegratorRTWStateStorageClass=Auto  FilterContinuousStateAttributes=''  FilterStateMustResolveToSignalObject=off  FilterRTWStateStorageClass=Auto  ParallelPVariant=Passthrough  IdealPVariant=InternalParameters  IVariant=InternalParameters  DVariant=Disabled  IntegratorVariant=Continuous  SatVariant=Enabled  AWVariant=Passthrough  PCopyVariant=Disabled  TRVariant=Disabled  FdbkBlocksVariant=Forward  IdealPFdbkVariant=Disabled  SatFdbkVariant=Disabled  DerivativeFilterVariant=Disabled  NVariant=Disabled  NCopyVariant=Disabled_SignalSpec  FilterICVariant=Disabled  IntegratorICVariant=InternalICs  ExternalResetVariant=ExternalReset  TRSumVariant=Passthrough  SumFdbkVariant=Disabled  SumVariant=Sum_PI  TsampFilterVariant=InternalTs  TsampNgainVariant=Passthrough  TsampIntegralVariant=Disabled_SignalSpec  ExternalSaturationOutDataTypeStr=Inherit: Same as second input
  Subsystem1 : $bdroot/SVR Control/Subsystem1  SystemSampleTime=-1  VariantActivationTime=update diagram  Latency=0  AutoFrameSizeCalculation=off
  Subsystem2 : $bdroot/SVR Control/Subsystem2  SystemSampleTime=-1  VariantActivationTime=update diagram  Latency=0  AutoFrameSizeCalculation=off
  Subtract : Sum  Inputs=+-
  Switch : Switch  Criteria=u2 > Threshold  SaturateOnIntegerOverflow=off  InputSameDT=off
  Switch1 : Switch  Criteria=u2 > Threshold  SaturateOnIntegerOverflow=off  InputSameDT=off
  Switch2 : Switch  Criteria=u2 > Threshold  SaturateOnIntegerOverflow=off  InputSameDT=off
  Unit Delay2 : UnitDelay  SampleTime=-1  HasFrameUpgradeWarning=on
  wires:
  Subsystem1/1 -> Switch/2
  Switch1/1 -> Switch/1, Subtract/1
  [UVV] -> Subsystem1/1, Switch/3
  Subtract/1 -> PID Controller1/1  "V(t)"
  Switch/1 -> Subtract/2
  Constant/1 -> Switch1/3
  Constant1/1 -> OR/1
  UVV(t)/1 -> Switch1/2, IsZero1/1, Switch1/1
  IsZero1/1 -> OR/2
  Switch2/1 -> Data Store Write/1
  K_uvv/1 -> Switch2/3
  OR/1 -> PID Controller1/2, MATLAB Function/Trigger, Unit Delay2/1, Subsystem2/2
  PID Controller1/1 -> Subsystem2/1
  Unit Delay2/1 -> Switch2/2
  Subsystem2/1 -> MATLAB Function/1(u), Switch2/1

== system Vessel/V_ed ==
  V(t) : Inport
  Data Store Read : DataStoreRead  Commented=on  DataStoreName=T  IndexOptions=Index vector (dialog)  Indices=1  OutputSizes=1
  Gain : Gain  Commented=on  Gain=0.5
  MinMax Running Resettable1 : simulink/Math Operations/MinMax Running Resettable  Function=max  vinit=0
      settings: AttributesFormatString=%<vinit>
  Pulse Generator1 : DiscretePulseGenerator  PulseType=Time based  TimeSource=Use external signal  Period=100  PulseWidth=1e-3
  Pulse Generator2 : DiscretePulseGenerator  PulseType=Time based  TimeSource=Use external signal  Period=100  PulseWidth=1e-3  PhaseDelay=0.2
  Sample and Hold1 : dspsigops/Sample and Hold  trig=Rising edge  initCond=0  latchinput=on
  Variable Transport Delay : VariableTransportDelay  Commented=on  VariableDelayType=Variable transport delay  MaximumDelay=10
  v_ed : Outport
  wires:
  V(t)/1 -> MinMax Running Resettable1/1
  Sample and Hold1/1 -> v_ed/1
  MinMax Running Resettable1/1 -> Sample and Hold1/1
  [t_b] -> Pulse Generator2/1, Pulse Generator1/1
  Data Store Read/1 -> Gain/1
  Pulse Generator1/1 -> MinMax Running Resettable1/2
  Gain/1 -> Variable Transport Delay/2
  Pulse Generator2/1 -> Sample and Hold1/Trigger

== system Vessel/V_ed calculation (old) ==
  V(t) : Inport
  Constant : Constant  Value=0.001
  Data Store Read : DataStoreRead  DataStoreName=T  IndexOptions=Index vector (dialog)  Indices=1  OutputSizes=1
  Gain : Gain  Gain=-1
  Memory : Memory
  MinMax Running Resettable : simulink/Math Operations/MinMax Running Resettable  Function=max  vinit=0
      settings: AttributesFormatString=%<vinit>
  Switch1 : Switch  SaturateOnIntegerOverflow=off  InputSameDT=off
  Transport Delay : TransportDelay  DelayTime=t_delay
  Variable Pulse Generator : VariablePulseGenerator  AllowZeroPulseWidth=on  RunAtFixedTimeIntervals=on  SampleTime=Ts
  v_ed : Outport
  wires:
  Switch1/1 -> v_ed/1, Memory/1
  MinMax Running Resettable/1 -> Switch1/3
  Memory/1 -> Switch1/1
  V(t)/1 -> MinMax Running Resettable/1
  Constant/1 -> Variable Pulse Generator/1
  Data Store Read/1 -> Variable Pulse Generator/2
  Transport Delay/1 -> MinMax Running Resettable/2
  Variable Pulse Generator/1 -> Gain/1, Transport Delay/1
  Gain/1 -> Switch1/2

== system Vessel/V_ed_new ==
  V(t) : Inport
  Data Store Read : DataStoreRead  DataStoreName=T  IndexOptions=Index vector (dialog)  Indices=1  OutputSizes=1
  IsPositive : simulink/Logic and Bit Operations/Compare To Zero  relop=>  OutDataTypeStr=boolean
  Product : Product
  Pulse Generator3 : DiscretePulseGenerator  PulseType=Time based  TimeSource=Use external signal  Period=100  PulseWidth=1e-3
  Sample and Hold1 : dspsigops/Sample and Hold  trig=Rising edge  initCond=V_0  latchinput=on
  Subsystem2 : $bdroot/Time varying elastance1/Subsystem/Subsystem2  SystemSampleTime=-1  VariantActivationTime=update diagram  Latency=0  AutoFrameSizeCalculation=off
  Subtract : Sum  Inputs=+-
  v_ed : Outport
  wires:
  Pulse Generator3/1 -> Sample and Hold1/Trigger
  V(t)/1 -> Sample and Hold1/1
  Subsystem2/1 -> Subtract/2
  [t_b] -> Subtract/1
  IsPositive/1 -> Product/2
  Product/1 -> Pulse Generator3/1
  Subtract/1 -> IsPositive/1, Product/1
  Data Store Read/1 -> Subsystem2/1
  Sample and Hold1/1 -> v_ed/1

== system Vessel/Valve1 ==
  note: The bernoulli resistance and the inductance really affect the behaviour of the whole system!! No the bernoulli resistance has been divide by 100, which seems to generate physiological outputs. Howver the peak flow is high, prolly due to the low amount of blood in the system.
  P_Input : Inport
  P_Output : Inport  Port=2
  Effective Area : Subsystem
  Integrator : Integrator  LimitOutput=on  UpperSaturationLimit=Q_max  LowerSaturationLimit=Q_min
  MATLAB Function : MATLAB Function  Commented=on  TreatAsAtomicUnit=on
  Product : Product  Inputs=3
  Product1 : Product  Inputs=*/
  Saturation1 : Saturate  UpperLimit=100  LowerLimit=0.0004
  Subsystem : Subsystem
  Sum : Sum  Inputs=+-
  Sum1 : Sum  Inputs=+-
  |Q_Input| : Abs  SaturateOnIntegerOverflow=off
  Q_Input : Outport
  A_eff(t) : Outport  Port=2
  wires:
  Subsystem/1(B_Valve) -> Saturation1/1  "B_Valve"
  Product1/1 -> Integrator/1  "Q_Input'"
  |Q_Input|/1 -> Product/1
  Integrator/1 -> Product/3, |Q_Input|/1, Q_Input/1  "Q_Input"
  Sum1/1 -> Effective Area/1("ΔP  "), Sum/1  "ΔP"
  Subsystem/2(L_Valve) -> Product1/2  "L_Valve"
  Product/1 -> Sum/2
  P_Input/1 -> Sum1/1
  P_Output/1 -> Sum1/2
  Sum/1 -> Product1/1
  Saturation1/1 -> Product/2
  Effective Area/1(A_eff(t)) -> A_eff(t)/1, Subsystem/1(A_eff(t))

== system Vessel/Vascular Impedance ==
  V(t) : Inport
  Inductance : $bdroot/Inductance  SystemSampleTime=-1  VariantActivationTime=update diagram  Latency=0  AutoFrameSizeCalculation=off
  Radius : $bdroot/Radius  SystemSampleTime=-1  VariantActivationTime=update diagram  Latency=0  AutoFrameSizeCalculation=off
  Resistance : $bdroot/Resistance  SystemSampleTime=-1  VariantActivationTime=update diagram  Latency=0  AutoFrameSizeCalculation=off
  L(t) : Outport
  R(t) : Outport  Port=2
  wires:
  Radius/1 -> Inductance/1, Resistance/1  "r(t)"
  Resistance/1 -> R(t)/1
  V(t)/1 -> Radius/1
  Inductance/1 -> L(t)/1

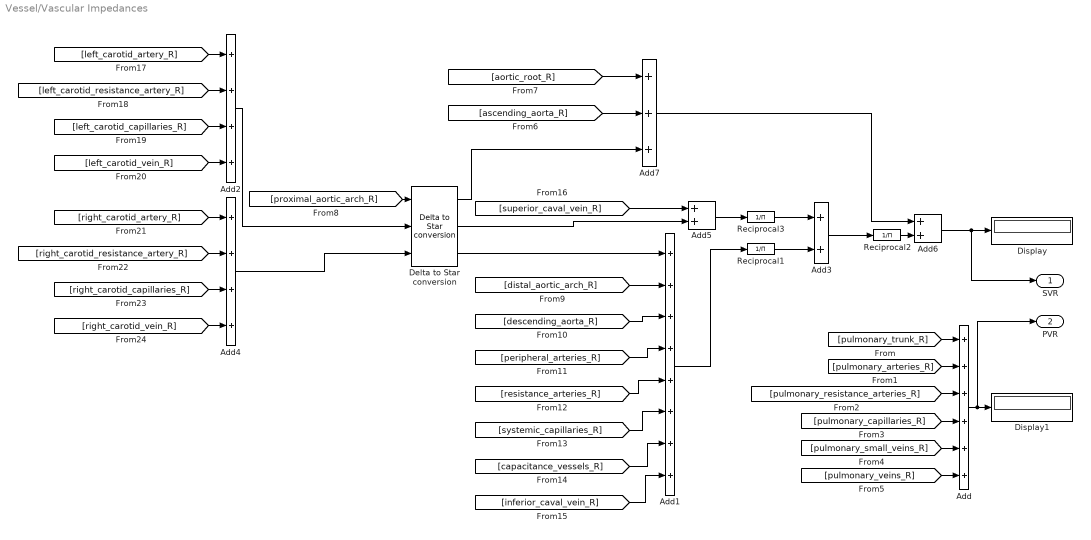
== system Vessel/Vascular Impedances ==
  Add : Sum  Inputs=6
  Add1 : Sum  Inputs=8
  Add2 : Sum  Inputs=4
  Add3 : Sum  Inputs=2
  Add4 : Sum  Inputs=4
  Add5 : Sum
  Add6 : Sum
  Add7 : Sum  Inputs=3
  Delta to Star conversion : $bdroot/Delta to Star conversion  SystemSampleTime=-1  VariantActivationTime=update diagram  Latency=0  AutoFrameSizeCalculation=off
  Display : Display
  Display1 : Display
  Reciprocal1 : Product  Inputs=/
  Reciprocal2 : Product  Inputs=/
  Reciprocal3 : Product  Inputs=/
  SVR : Outport
  PVR : Outport  Port=2
  wires:
  [pulmonary_small_veins_R] -> Add/5
  [pulmonary_capillaries_R] -> Add/4
  [pulmonary_resistance_arteries_R] -> Add/3
  [pulmonary_arteries_R] -> Add/2
  [pulmonary_trunk_R] -> Add/1
  [pulmonary_veins_R] -> Add/6
  [superior_caval_vein_R] -> Add5/1
  [left_carotid_artery_R] -> Add2/1
  [left_carotid_capillaries_R] -> Add2/3
  [left_carotid_resistance_artery_R] -> Add2/2
  [left_carotid_vein_R] -> Add2/4
  [right_carotid_artery_R] -> Add4/1
  [right_carotid_capillaries_R] -> Add4/3
  [right_carotid_resistance_artery_R] -> Add4/2
  [right_carotid_vein_R] -> Add4/4
  Add4/1 -> Delta to Star conversion/3
  Add3/1 -> Reciprocal2/1
  Reciprocal1/1 -> Add3/2
  Add6/1 -> SVR/1, Display/1
  Add5/1 -> Reciprocal3/1
  Reciprocal3/1 -> Add3/1
  [proximal_aortic_arch_R] -> Delta to Star conversion/1
  Add2/1 -> Delta to Star conversion/2
  [aortic_root_R] -> Add7/1
  [ascending_aorta_R] -> Add7/2
  Delta to Star conversion/1 -> Add7/3
  [distal_aortic_arch_R] -> Add1/2
  [descending_aorta_R] -> Add1/3
  [peripheral_arteries_R] -> Add1/4
  [resistance_arteries_R] -> Add1/5
  [systemic_capillaries_R] -> Add1/6
  [capacitance_vessels_R] -> Add1/7
  [inferior_caval_vein_R] -> Add1/8
  Add1/1 -> Reciprocal1/1
  Reciprocal2/1 -> Add6/2
  Add7/1 -> Add6/1
  Delta to Star conversion/2 -> Add5/2
  Delta to Star conversion/3 -> Add1/1
  Add/1 -> PVR/1, Display1/1

== system Vessel/Vessel (L-inverted) ==
  Q_Output : Inport
  P_Input : Inport  Port=2
  " " : Sum  Inputs=-+-
  "   " : Sum  Inputs=-+
  Add : Sum  Inputs=+-
  Add1 : Sum
  Constant1 : Constant  Value=V0
  Delay : Delay  InitialCondition=P0  UseCircularBuffer=on
  Gain UVV : $bdroot/Gain UVV  SystemSampleTime=-1  VariantActivationTime=update diagram  Latency=0  AutoFrameSizeCalculation=off
  IC : InitialCondition  Value=P0
  IC1 : InitialCondition  Value=0
  Integrator : Integrator  InitialConditionSource=external  LimitOutput=on  LowerSaturationLimit=0  ContinuousStateAttributes='Volume'
  Integrator2 : Integrator  LimitOutput=on  UpperSaturationLimit=4000  LowerSaturationLimit=-4000  ContinuousStateAttributes='Flow'
  Omega : $bdroot/Omega  SystemSampleTime=-1  VariantActivationTime=update diagram  Latency=0  AutoFrameSizeCalculation=off
  Product2 : Product
  Product3 : Product  Inputs=*/
  Product4 : Product
  Transmural Pressure : $bdroot/Transmural Pressure  SystemSampleTime=-1  VariantActivationTime=update diagram  Latency=0  AutoFrameSizeCalculation=off
  Vascular Impedance : $bdroot/Vascular Impedance  SystemSampleTime=-1  VariantActivationTime=update diagram  Latency=0  AutoFrameSizeCalculation=off
  Q_Input : Outport
  P_Output : Outport  Port=2  Unit=mmHg
  V(t) : Outport  Port=3
  R : Outport  Port=4
  wires:
  Product3/1 -> Integrator2/1  "Q_Input'"
  Integrator/1 -> Add/1, V(t)/1  "V(t)"
  Add/1 -> Transmural Pressure/1  "V-V0"
  Product2/1 -> " "/3  "P_R"
  " "/1 -> Product3/1
  Add1/1 -> " "/1, IC/1
  Transmural Pressure/1 -> Add1/1  "P_c"
  Product4/1 -> Add1/2  "P_Ω"
  Omega/1 -> Product4/1  "Ω"
  P_Input/1 -> " "/2
  Integrator2/1 -> Q_Input/1, "   "/2, Product2/1  "Q_Input"
  Constant1/1 -> Gain UVV/1
  "   "/1 -> IC1/1  "V(t)'"
  Vascular Impedance/1 -> Product3/2
  IC1/1 -> Product4/2, Integrator/1
  Q_Output/1 -> "   "/1
  IC/1 -> Delay/1
  Delay/1 -> P_Output/1
  Vascular Impedance/2 -> R/1, Product2/2
  Gain UVV/1 -> Integrator/2, Vascular Impedance/1, Add/2

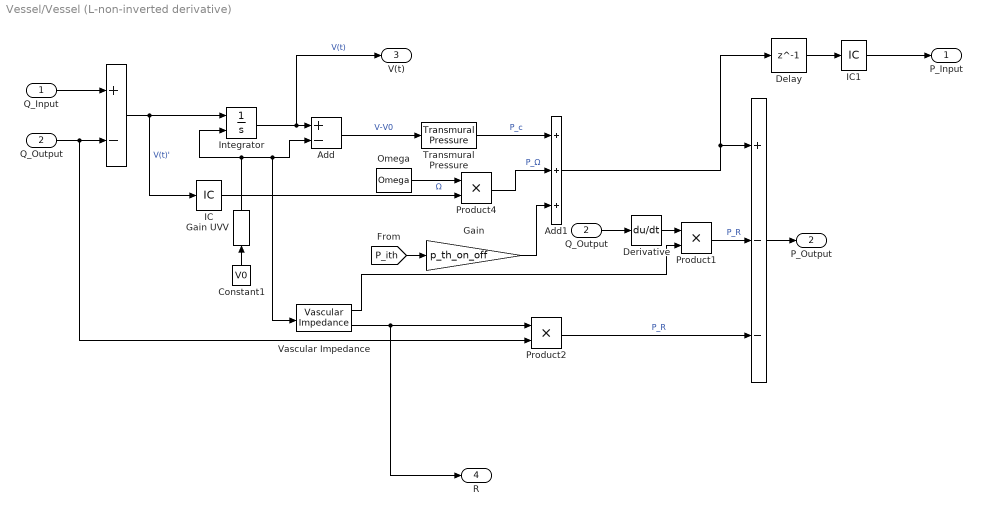
== system Vessel/Vessel (L-non-inverted derivative) ==
  Q_Input : Inport
  Q_Output : Inport  Port=2
  " " : Sum  Inputs=+--
  "   " : Sum  Inputs=+-
  Add : Sum  Inputs=+-
  Add1 : Sum  Inputs=+++
  Constant1 : Constant  Value=V0
  Delay : Delay  DelayLength=1  InitialCondition=P0
  Derivative : Derivative
  Gain : Gain  Gain=p_th_on_off
  Gain UVV : $bdroot/Gain UVV  SystemSampleTime=-1  VariantActivationTime=update diagram  Latency=0  AutoFrameSizeCalculation=off
  IC : InitialCondition  Value=0
  IC1 : InitialCondition  Value=P0
  Integrator : Integrator  InitialConditionSource=external  LimitOutput=on  LowerSaturationLimit=0  ContinuousStateAttributes='Volume'
  Omega : $bdroot/Omega  SystemSampleTime=-1  VariantActivationTime=update diagram  Latency=0  AutoFrameSizeCalculation=off
  Product1 : Product
  Product2 : Product
  Product4 : Product
  "Q_Output " : InportShadow  Port=2
  Transmural Pressure : $bdroot/Transmural Pressure  SystemSampleTime=-1  VariantActivationTime=update diagram  Latency=0  AutoFrameSizeCalculation=off
  Vascular Impedance : $bdroot/Vascular Impedance  SystemSampleTime=-1  VariantActivationTime=update diagram  Latency=0  AutoFrameSizeCalculation=off
  P_Input : Outport
  P_Output : Outport  Port=2
  V(t) : Outport  Port=3
  R : Outport  Port=4
  wires:
  Delay/1 -> IC1/1
  IC1/1 -> P_Input/1
  IC/1 -> Product4/2
  Gain/1 -> Add1/3
  [P_ith] -> Gain/1
  Vascular Impedance/1 -> Product1/2
  "   "/1 -> Integrator/1, IC/1  "V(t)'"
  Integrator/1 -> Add/1, V(t)/1  "V(t)"
  Add/1 -> Transmural Pressure/1  "V-V0"
  Product2/1 -> " "/3  "P_R"
  Add1/1 -> " "/1, Delay/1
  Transmural Pressure/1 -> Add1/1  "P_c"
  Q_Input/1 -> "   "/1
  Product4/1 -> Add1/2  "P_Ω"
  Omega/1 -> Product4/1  "Ω"
  Constant1/1 -> Gain UVV/1
  Q_Output/1 -> Product2/2, "   "/2
  "Q_Output "/1 -> Derivative/1
  Derivative/1 -> Product1/1
  Product1/1 -> " "/2  "P_R"
  " "/1 -> P_Output/1
  Vascular Impedance/2 -> R/1, Product2/1
  Gain UVV/1 -> Vascular Impedance/1, Add/2, Integrator/2
